simulink model "RefModel_SignalFault"  (R2020a)
settings: Solver=ode1  StartTime=0.0  StopTime=100  FixedStep=1/sensorFs.imuUpdateFs  MaxStep=Ts  RelTol=1e-3
undefined symbols (not defined in the file or in its folder): sensorFs
libraries: simulink x11
settings Model: Creator=sl  LastModifiedBy=sl
settings OptimizationCC: DefaultParameterBehavior=Inlined  EnhancedBackFolding=on  PassReuseOutputArgsAs=Individual arguments  ZeroExternalMemoryAtStartup=off  ZeroInternalMemoryAtStartup=off  OptimizeBlockOrder=speed  DifferentSizesBufferReuse=on  OptimizationCustomize=off  EfficientTunableParamExpr=on
settings DebuggingCC: ParameterTunabilityLossMsg=error
settings HardwareCC: ProdBitPerPointer=32  ProdBitPerSizeT=32  ProdBitPerPtrDiffT=32  ProdLargestAtomicInteger=Long  ProdLargestAtomicFloat=Double  ProdWordSize=32  ProdHWDeviceType=ARM Compatible->ARM Cortex
settings SFSimCC: MATLABDynamicMemAlloc=off
settings RTWCC: SystemTargetFile=ert.tlc  GenCodeOnly=on  PackageGeneratedCodeAndArtifacts=on  TemplateMakefile=ert_default_tmf  GenerateReport=on  IncludeHyperlinkInReport=on  LaunchReport=on  GenerateTraceInfo=on  GenerateTraceReport=on  GenerateTraceReportSl=on  GenerateTraceReportSf=on  GenerateTraceReportEml=on
settings CodeAppCC: ForceParamTrailComments=on  IgnoreCustomStorageClasses=off  OperatorAnnotations=on  SimulinkDataObjDesc=on  SFDataObjDesc=on  InsertBlockDesc=on
settings ERTTargetCC: TargetLangStandard=C99 (ISO)  CodeReplacementLibrary=ARM Cortex-M (Optimized)  GenerateSampleERTMain=on  SupportVariableSizeSignals=on  InlinedParameterPlacement=NonHierarchical  ERTCustomFileTemplate=example_file_process.tlc  ERTFilePackagingFormat=Compact

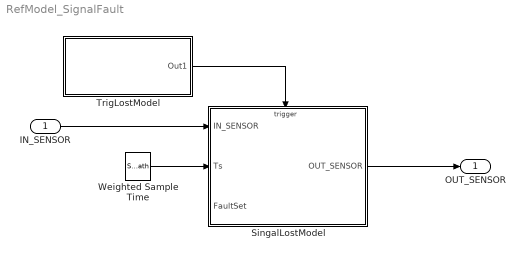
== system RefModel_SignalFault ==
  IN_SENSOR : Inport  OutDataTypeStr=Bus: BUS_SENSOR  BusOutputAsStruct=on
  SingalLostModel : Stateflow chart  TreatAsAtomicUnit=on
  TrigLostModel : Subsystem
  Weighted Sample Time : SampleTimeMath  TsampMathOp=Ts Only
  OUT_SENSOR : Outport  OutDataTypeStr=Bus: BUS_SENSOR  BusOutputAsStruct=on
  wires:
  IN_SENSOR/1 -> SingalLostModel/1(IN_SENSOR)
  SingalLostModel/1(OUT_SENSOR) -> OUT_SENSOR/1
  TrigLostModel/1(Out1) -> SingalLostModel/Trigger
  Weighted Sample Time/1 -> SingalLostModel/2(Ts)
  ? -> SingalLostModel/3(FaultSet)

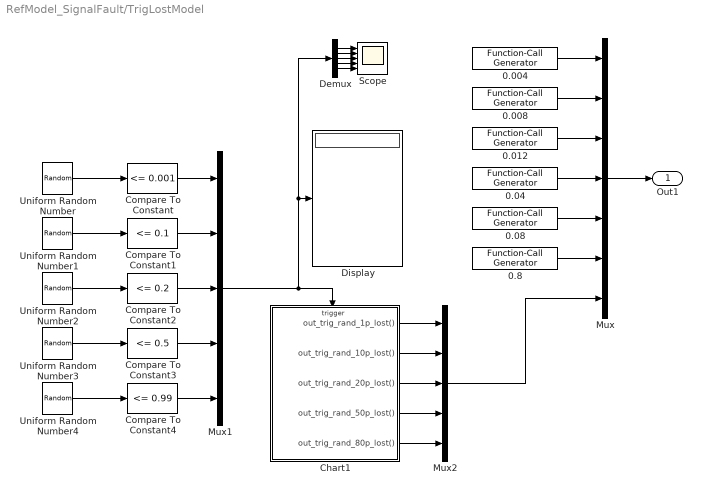
== system RefModel_SignalFault/TrigLostModel ==
  0.004 : simulink/Ports & Subsystems/Function-Call Generator  sample_time=0.004  numberOfIterations=1
  0.008 : simulink/Ports & Subsystems/Function-Call Generator  sample_time=0.008  numberOfIterations=1
  0.012 : simulink/Ports & Subsystems/Function-Call Generator  sample_time=0.012  numberOfIterations=1
  0.04 : simulink/Ports & Subsystems/Function-Call Generator  sample_time=0.04  numberOfIterations=1
  0.08 : simulink/Ports & Subsystems/Function-Call Generator  sample_time=0.08  numberOfIterations=1
  0.8 : simulink/Ports & Subsystems/Function-Call Generator  sample_time=0.8  numberOfIterations=1
  Chart1 : Stateflow chart  TreatAsAtomicUnit=on
  Compare To Constant : simulink/Logic and Bit Operations/Compare To Constant  relop=<=  const=0.001  OutDataTypeStr=boolean
  Compare To Constant1 : simulink/Logic and Bit Operations/Compare To Constant  relop=<=  const=0.1  OutDataTypeStr=boolean
  Compare To Constant2 : simulink/Logic and Bit Operations/Compare To Constant  relop=<=  const=0.2  OutDataTypeStr=boolean
  Compare To Constant3 : simulink/Logic and Bit Operations/Compare To Constant  relop=<=  const=0.5  OutDataTypeStr=boolean
  Compare To Constant4 : simulink/Logic and Bit Operations/Compare To Constant  relop=<=  const=0.99  OutDataTypeStr=boolean
  Demux : Demux  Outputs=5
  Display : Display
  Mux : Mux  Inputs=7
  Mux1 : Mux  Inputs=5
  Mux2 : Mux  Inputs=5
  Scope : Scope  NumInputPorts=5
  Uniform Random Number : UniformRandomNumber  Minimum=0  SampleTime=1/sensorFs.imuUpdateFs
  Uniform Random Number1 : UniformRandomNumber  Minimum=0  Seed=1  SampleTime=1/sensorFs.imuUpdateFs
  Uniform Random Number2 : UniformRandomNumber  Minimum=0  Seed=2  SampleTime=1/sensorFs.imuUpdateFs
  Uniform Random Number3 : UniformRandomNumber  Minimum=0  Seed=3  SampleTime=1/sensorFs.imuUpdateFs
  Uniform Random Number4 : UniformRandomNumber  Minimum=0  Seed=4  SampleTime=1/sensorFs.imuUpdateFs
  Out1 : Outport
  wires:
  0.8/1 -> Mux/6
  Chart1/3(out_trig_rand_20p_lost()) -> Mux2/3
  Compare To Constant1/1 -> Mux1/2
  Compare To Constant3/1 -> Mux1/4
  Compare To Constant4/1 -> Mux1/5
  Chart1/1(out_trig_rand_1p_lost()) -> Mux2/1
  0.08/1 -> Mux/5
  Mux/1 -> Out1/1
  Uniform Random Number3/1 -> Compare To Constant3/1
  0.004/1 -> Mux/1
  Mux1/1 -> Chart1/Trigger, Demux/1, Display/1
  Mux2/1 -> Mux/7
  Uniform Random Number4/1 -> Compare To Constant4/1
  Demux/1 -> Scope/1
  Compare To Constant/1 -> Mux1/1
  0.04/1 -> Mux/4
  Compare To Constant2/1 -> Mux1/3
  Uniform Random Number2/1 -> Compare To Constant2/1
  0.012/1 -> Mux/3
  Uniform Random Number/1 -> Compare To Constant/1
  Uniform Random Number1/1 -> Compare To Constant1/1
  Chart1/2(out_trig_rand_10p_lost()) -> Mux2/2
  Chart1/4(out_trig_rand_50p_lost()) -> Mux2/4
  Demux/5 -> Scope/5
  Chart1/5(out_trig_rand_80p_lost()) -> Mux2/5
  0.008/1 -> Mux/2
  Demux/2 -> Scope/2
  Demux/4 -> Scope/4
  Demux/3 -> Scope/3

== stateflow chart RefModel_SignalFault/TrigLostModel/Chart1 ==
  state TRIG_1Percent_LOST [parallel]
    settings: executionOrder=1
    state Normal
    state Normal1
    (default) -> TRIG_1Percent_LOST.Normal
    TRIG_1Percent_LOST.Normal1 -> TRIG_1Percent_LOST.Normal : trig_rand_1p_lost
        | {send(out_trig_rand_1p_lost)}
    TRIG_1Percent_LOST.Normal -> TRIG_1Percent_LOST.Normal1 : trig_rand_1p_lost
        | {send(out_trig_rand_1p_lost)}
  state TRIG_10Percent_LOST [parallel]
    settings: executionOrder=2
    state Normal
    state Normal1
    (default) -> TRIG_10Percent_LOST.Normal
    TRIG_10Percent_LOST.Normal1 -> TRIG_10Percent_LOST.Normal : trig_rand_10p_lost
        | {send(out_trig_rand_10p_lost)}
    TRIG_10Percent_LOST.Normal -> TRIG_10Percent_LOST.Normal1 : trig_rand_10p_lost
        | {send(out_trig_rand_10p_lost)}
  state TRIG_20Percent_LOST [parallel]
    settings: executionOrder=3
    state Normal
    state Normal1
    (default) -> TRIG_20Percent_LOST.Normal
    TRIG_20Percent_LOST.Normal1 -> TRIG_20Percent_LOST.Normal : trig_rand_20p_lost
        | {send(out_trig_rand_20p_lost)}
    TRIG_20Percent_LOST.Normal -> TRIG_20Percent_LOST.Normal1 : trig_rand_20p_lost
        | {send(out_trig_rand_20p_lost)}
  state TRIG_50Percent_LOST [parallel]
    settings: executionOrder=4
    state Normal
    state Normal1
    (default) -> TRIG_50Percent_LOST.Normal
    TRIG_50Percent_LOST.Normal1 -> TRIG_50Percent_LOST.Normal : trig_rand_50p_lost
        | {send(out_trig_rand_50p_lost)}
    TRIG_50Percent_LOST.Normal -> TRIG_50Percent_LOST.Normal1 : trig_rand_50p_lost
        | {send(out_trig_rand_50p_lost)}
  state TRIG_80Percent_LOST [parallel]
    settings: executionOrder=5
    state Normal
    state Normal1
    (default) -> TRIG_80Percent_LOST.Normal
    TRIG_80Percent_LOST.Normal1 -> TRIG_80Percent_LOST.Normal : trig_rand_80p_lost
        | {send(out_trig_rand_80p_lost)}
    TRIG_80Percent_LOST.Normal -> TRIG_80Percent_LOST.Normal1 : trig_rand_80p_lost
        | {send(out_trig_rand_80p_lost)}
  events: trig_rand_1p_lost input RISING_EDGE_EVENT; trig_rand_10p_lost input RISING_EDGE_EVENT; trig_rand_20p_lost input RISING_EDGE_EVENT; trig_rand_50p_lost input RISING_EDGE_EVENT; trig_rand_80p_lost input RISING_EDGE_EVENT; out_trig_rand_1p_lost output FUNCTION_CALL_EVENT; out_trig_rand_10p_lost output FUNCTION_CALL_EVENT; out_trig_rand_20p_lost output FUNCTION_CALL_EVENT; out_trig_rand_50p_lost output FUNCTION_CALL_EVENT; out_trig_rand_80p_lost output FUNCTION_CALL_EVENT

== stateflow chart RefModel_SignalFault/SingalLostModel ==
  settings: executeAtInitialization=1
  state IMU1 [parallel]
    settings: executionOrder=1
    state Normal
      en:
      idx = idx + 1;
      du:
      OUT_SENSOR.IMU1 = IN_SENSOR.IMU1;
    state Lost
      % Keep Last Value
      en:
      du:
    (default) -> IMU1.Normal : {idx = 0;}
    IMU1.Lost -> IMU1.Normal : after(idx,sec)
    IMU1.Normal -> IMU1.Lost : trig_200_Ts
  state IMU2 [parallel]
    settings: executionOrder=2
    state Normal
      du:
      OUT_SENSOR.IMU2 = IN_SENSOR.IMU2;
    state Lost
      % Keep Last Value
    (default) -> IMU2.Normal
    IMU2.Lost -> IMU2.Normal : after(2,sec)
    IMU2.Normal -> IMU2.Lost : trig_200_Ts
  state IMU3 [parallel]
    settings: executionOrder=3
    state Normal
      du:
      OUT_SENSOR.IMU3 = IN_SENSOR.IMU3;
    state Lost
      % Keep Last Value
    (default) -> IMU3.Normal
    IMU3.Lost -> IMU3.Normal : after(2,sec)
    IMU3.Normal -> IMU3.Lost : trig_rand_10p_lost
  state Others [parallel]
    settings: executionOrder=4
    state Normal
      du:
      OUT_SENSOR.mag1 = IN_SENSOR.mag1;
      OUT_SENSOR.mag2 = IN_SENSOR.mag2;
      OUT_SENSOR.time = IN_SENSOR.time;
      OUT_SENSOR.um482 = IN_SENSOR.um482;
      OUT_SENSOR.airspeed1 = IN_SENSOR.airspeed1;
      OUT_SENSOR.radar1 = IN_SENSOR.radar1;
      OUT_SENSOR.baro1 = IN_SENSOR.baro1;
    state Lost
      % Keep Last Value
      en:
      du:
    (default) -> Others.Normal
    Others.Lost -> Others.Normal : after(2,sec)
  data: IN_SENSOR input Bus: BUS_SENSOR; OUT_SENSOR output Bus: BUS_SENSOR; Ts input; idx local; FaultSet input
  events: trig_1_Ts input FUNCTION_CALL_EVENT; trig_2_Ts input FUNCTION_CALL_EVENT; trig_3_Ts input FUNCTION_CALL_EVENT; trig_10_Ts input FUNCTION_CALL_EVENT; trig_20_Ts input FUNCTION_CALL_EVENT; trig_200_Ts input FUNCTION_CALL_EVENT; trig_rand_1p_lost input FUNCTION_CALL_EVENT; trig_rand_10p_lost input FUNCTION_CALL_EVENT; trig_rand_20p_lost input FUNCTION_CALL_EVENT; trig_rand_50p_lost input FUNCTION_CALL_EVENT; trig_rand_80p_lost input FUNCTION_CALL_EVENT
